simulink model "Motor_model"  (R2023a)
settings: Solver=VariableStepAuto  StartTime=0.0  StopTime=table.Time_ms_(end)/1000  RelTol=1e-3
InitFcn:
  | % Motor Constants
  | noLoadCurrent = 2.1; % Amp
  | noLoadSpeed = 5600; % RPM
  | noLoadSpeed_rad = noLoadSpeed * 2*pi / 60; % rad/s
  | Km = 0.04025; % Nm / Amp
  | 
  | BM = 0.1 * noLoadCurrent * Km / noLoadSpeed_rad; % Nms
  | 
  | R_terminal = 0.3 % 0.19; % Ohms
  | L_terminal = 188e-6; %Henrys
  | 
  | % System Constants
  | JM = 6*612 / 1000 / 100^2; %kg*m^2
  | 
  | s = tf('s');
  | 
  | Ym = 1 / (JM * s + BM);
  | rad_sec_to_rpm = 60/(2*pi);
undefined symbols (not defined in the file): current_limit
libraries: cstblocks x1
settings Model: Creator=trent  LastModifiedBy=andre
settings OptimizationCC: ReuseModelBlockBuffer=off
settings DebuggingCC: UnconnectedInputMsg=warning  UnconnectedOutputMsg=warning  UnconnectedLineMsg=warning
settings ModelReferenceCC: EnableRefExpFcnMdlSchedulingChecks=on
settings RTWCC: DLArmComputeVersion=19.05

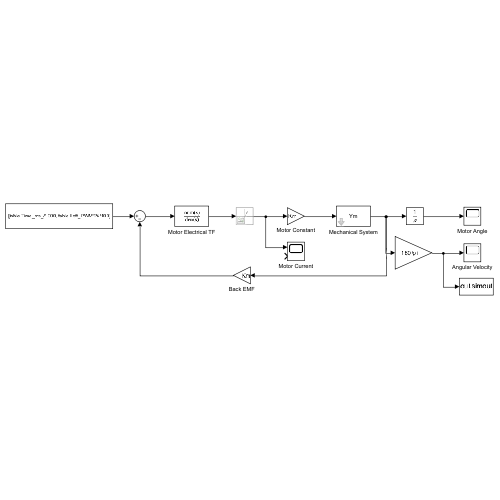
[thumbnail: Simulink's stored preview of the top-level diagram]
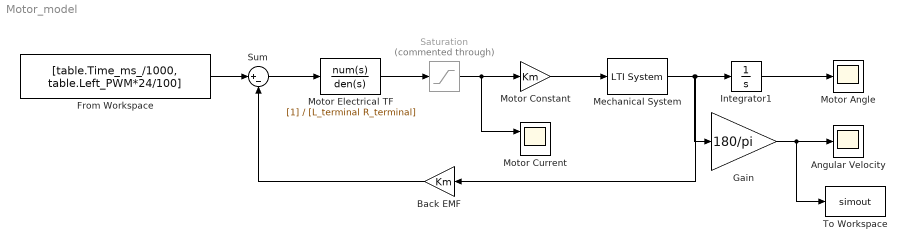
== system Motor_model ==
  Angular Velocity : Scope
  Back EMF : Gain  Gain=Km
  From Workspace : FromWorkspace  VariableName=[table.Time_ms_/1000, table.Left_PWM*24/100]
  Gain : Gain  Gain=180/pi
  Integrator1 : Integrator
  Mechanical System : cstblocks/LTI System  sys=Ym  IC=[]
  Motor Angle : Scope
  Motor Constant : Gain  Gain=Km
  Motor Current : Scope  NumInputPorts=2
  Motor Electrical TF : TransferFcn  Denominator=[L_terminal R_terminal]
  Saturation : Saturate  Commented=through  UpperLimit=current_limit  LowerLimit=-current_limit
  Sum : Sum  Inputs=|+-
  To Workspace : ToWorkspace  VariableName=simout  SaveFormat=Timeseries  SampleTime=-1
  wires:
  Mechanical System/1 -> Back EMF/1, Integrator1/1, Gain/1
  From Workspace/1 -> Sum/1
  Sum/1 -> Motor Electrical TF/1
  Motor Electrical TF/1 -> Saturation/1
  Back EMF/1 -> Sum/2
  Saturation/1 -> Motor Current/1, Motor Constant/1
  Motor Constant/1 -> Mechanical System/1
  Gain/1 -> Angular Velocity/1, To Workspace/1
  Integrator1/1 -> Motor Angle/1
